simulink library "Kitchen_Lib"  (R2023a)
settings: Solver=VariableStepAuto  StartTime=0.0  StopTime=10.0  RelTol=1e-3  EnableMultiTasking=on
undefined symbols (not defined in the file): Kitc_BusTyp_P, Kitc_BusTypSkyr_C, Kitc_ColrLedColrls_C, Kitc_ColrLedGrn_C, Kitc_ColrLedRed_C, Kitc_ColrLedYlw_C, Kitc_StDgnWtrTank_C, Kitc_StElecPlugScktOffByClmp50_P, Kitc_StsDlyBlink_C, Kitc_StsErrBlink_C, Kitc_StsFctAcvn_P, Kitc_StsInfoBlink_C, Kitc_StsKitchnOffAutoIgOff_P, Kitc_StsKitchnOffBySwt_P, Kitc_StsKitchnOffDoorLockd_P, Kitc_StsKitchnOffIgOff_P, Kitc_StsKitchnOffUv_P, Kitc_StsKitchnOnBySwt_P, Kitc_StsKitchnOnNVM_P, Kitc_StsLedOff_C, Kitc_StsLedOn_C, Kitc_StsLrgCnsAcv_P, Kitc_StTrfrAnSwtInstd_P, Kitc_StTrfrSwtInstd_P, Kitc_TiKitcRefgtrOffDly_P, Kitc_ULowrThdBat_C, Kitc_UUpprThdBat_C, Kitc_ValFalse_C, Kitc_ValPwmFreq2_C, Kitc_ValPwmFreq_C, Kitc_ValTrue_C
libraries: MAN_Library x50, E2E_Lib x3
(part 1 of 13)
settings Model: Creator=l4521  LastModifiedBy=u29w13
settings SolverCC: AlgebraicLoopSolver=TrustRegion
settings DataIOCC: LimitDataPoints=on  ReturnWorkspaceOutputs=off
settings OptimizationCC: LifeSpan=inf
settings DebuggingCC: UnconnectedInputMsg=warning  UnconnectedOutputMsg=warning  UnconnectedLineMsg=warning  AllowSymbolicDim=off  SFUnexpectedBacktrackingDiag=warning  SFNoUnconditionalDefaultTransitionDiag=warning  SFExecutionAtInitializationDiag=none  ArithmeticOperatorsInVariantConditions=warning
settings ModelReferenceCC: EnableRefExpFcnMdlSchedulingChecks=on  PropagateSignalLabelsOutOfModel=off
settings SFSimCC: SimUseLocalCustomCode=off  CustomCodeUndefinedFunction=UseInterfaceOnly
settings RTWCC: RTWUseLocalCustomCode=off
settings CodeAppCC: StateflowObjectComments=on
settings GRTTargetCC: TargetLangStandard=C89/C90 (ANSI)
settings ConfigComp: CovMetricSettings=dw  CovSaveCumulativeToWorkspaceVar=on  CovSaveSingleToWorkspaceVar=on  CovExternalEMLEnable=off

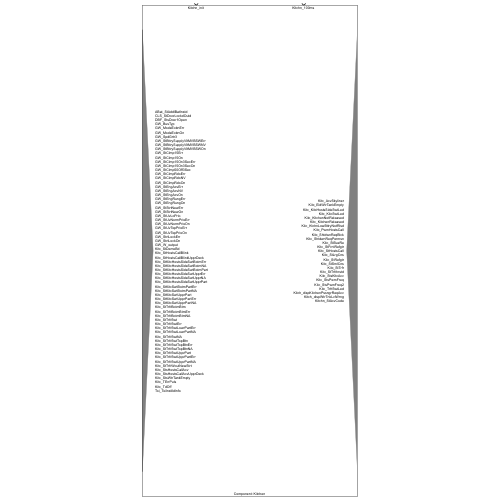
[thumbnail: Simulink's stored preview of the top-level diagram]
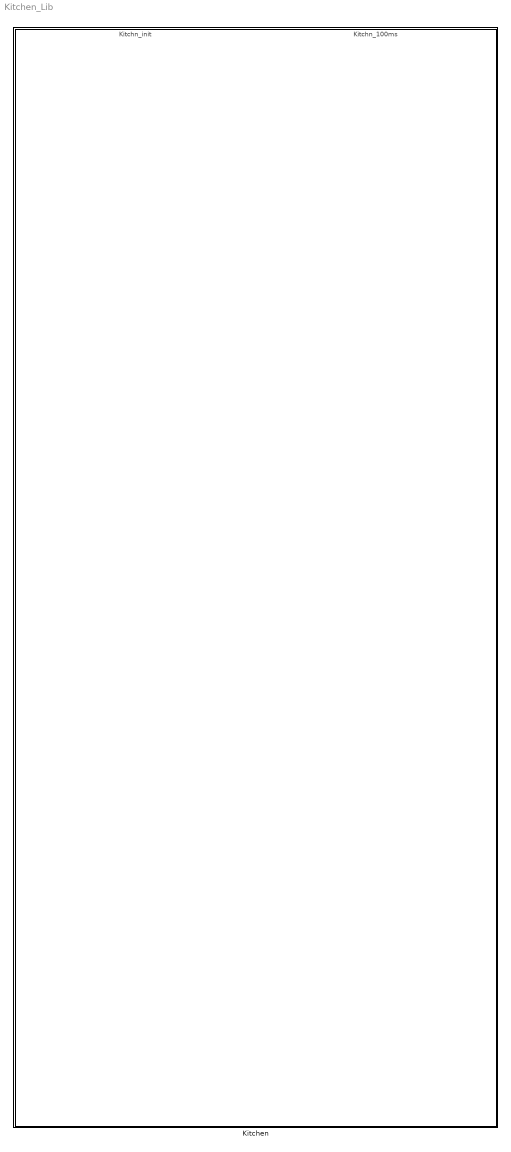
== system Kitchen_Lib ==
  Kitchen : Subsystem  mask(SW Component){}
      settings: MoveFcn=% evalin(get_param(bdroot, 'ModelWorkspace'), get_param(gcb, 'MaskInitialization'));
      mask Display:
      | % SWComponent_mask MaskDisplayStr for SWComponent block
      | %
      | %
      | 
      | % Copyright (c) AVL Software and Functions GmbH 2013
      | % $Revision: 1.42 $, $Date: 2019/08/13 04:53:27UTC $ by $Author: Urlhardt Franz RGB (urlhardf) $
      | 
      | % Calls:
      | 
      | % MaskVersion is used in sl_updateModelTemplate.
      | % $MaskVersion: 1$ % Version must be an integer
      | 
      | ShortName = get_param(gcb,'Name');
      | 
      | % Get inports of function cals
      | inports = find_system(gcb,'SearchDepth',1, 'FollowLinks','on', 'LookUnderMasks','all', 'BlockType','Inport');
      | FcArray = get_param(inports ,'Name');
      | FcXPos = ((1:6)-0.5)/length(FcArray);
      | FcArray(end+1:6) = {''};
      | 
      | % Look for other SW components 1 level below current block
      | SWComponents = find_system(gcb, 'SearchDepth',1, 'FollowLinks','on','LookUnderMasks','all','RegExp','on', 'MaskType','SW Component*');
      | % Remove current block from search results
      | SWComponents(ismember(SWComponents,gcb)) = [];
      | 
      | % A component is a level 3 component if there are no other SW Components below
      | isLevel3 = isempty(SWComponents);
      | 
      | 
      | if isLevel3
      |     % Level 3, Signals form ExtInp and ExtOut blocks
      |     ExtInp = find_system(gcb, 'SearchDepth',inf, 'FollowLinks','on','LookUnderMasks','all', 'MaskType','ExtInp ( AVLib TM )');
      |     ExtOut = find_system(gcb, 'SearchDepth',inf, 'FollowLinks','on','LookUnderMasks','all', 'MaskType','ExtOut ( AVLib TM )');
      | 
      |     Inputs = unique(get_param(ExtInp,'Signal'));
      |     Outputs = unique(get_param(ExtOut,'Signal'));
      | 
      |     %=> No AVLib
      |     if isempty(ExtInp) && isempty(ExtOut);
      |         DSRead = find_system(gcb, 'SearchDepth',2, 'FollowLinks','on','LookUnderMasks','all','BlockType','DataStoreRead');
      |         DSWrite = find_system(gcb, 'SearchDepth',2, 'FollowLinks','on','LookUnderMasks','all','BlockType','DataStoreWrite');
      |         Inputs = unique(get_param(DSRead,'DataStoreName'));
      |         Outputs = unique(get_param(DSWrite,'DataStoreName'));
      |     end
      | 
      |     InpArray = sprintf('%s\n',Inputs{:});
      | 
      |     % Remove last newline character
      |     if ~isempty(Inputs), InpArray(end) = []; end
      | 
      |     OutArray = sprintf('%s\n',Outputs{:});
      |     % Remove last newline character
      |     if ~isempty(Outputs),OutArray(end) = []; end
      | 
      | else
      |     % Level 1/Level 2, get other SWComponents
      |     Comps = get_param(SWComponents,'Name');
      |     CompsArray = sprintf('%s\n',Comps{:});
      |     if ~isempty(Comps), CompsArray(end) = []; end
      | end
      | 
      | 
      | %% Mask
      | % Triangles
      | patch( [0 0.05 0 nan 1 0.95 1],[0.95 0.5 0.05 nan 0.95 0.5 0.05], 0.5*[1 1 1] );
      | 
      | % Names of function calls
      | for i = 1:6
      |     text(FcXPos(i), 1, FcArray{i}, 'HorizontalAlignment','center',  'VerticalAlignment','top'  );
      | end
      | 
      | if isLevel3
      |     % Level 3, display signals of ExtInp and ExtOut blocks
      |     text(0.06, 0.5, InpArray, 'HorizontalAlignment','left',  'VerticalAlignment','middle' );
      |     text(0.94, 0.5, OutArray, 'HorizontalAlignment','right', 'VerticalAlignment','middle' );
      |     text(0.5, 0.0, ['Component: ',ShortName], 'HorizontalAlignment','center', 'VerticalAlignment','bottom' );
      | else
      |     % Level 1/ Level 2, display names of other components below mask
      |     text(0.5, 0.5, CompsArray, 'HorizontalAlignment','center',  'VerticalAlignment','middle' );
      |     text(0.5, 0.0, ['Component: ',ShortName], 'HorizontalAlignment','center', 'VerticalAlignment','bottom' );
      | end

== system Kitchen_Lib/Kitchen ==
  Kitchn_init : Inport
  Kitchn_100ms : Inport  Port=2
  100ms : Subsystem  TreatAsAtomicUnit=on
      settings: RTWSystemCode=Inline
  init : Subsystem  TreatAsAtomicUnit=on
      settings: RTWSystemCode=Inline
  wires:
  Kitchn_100ms/1 -> 100ms/Trigger  "Kitchn_100ms"
  Kitchn_init/1 -> init/Trigger  "Kitchn_init"

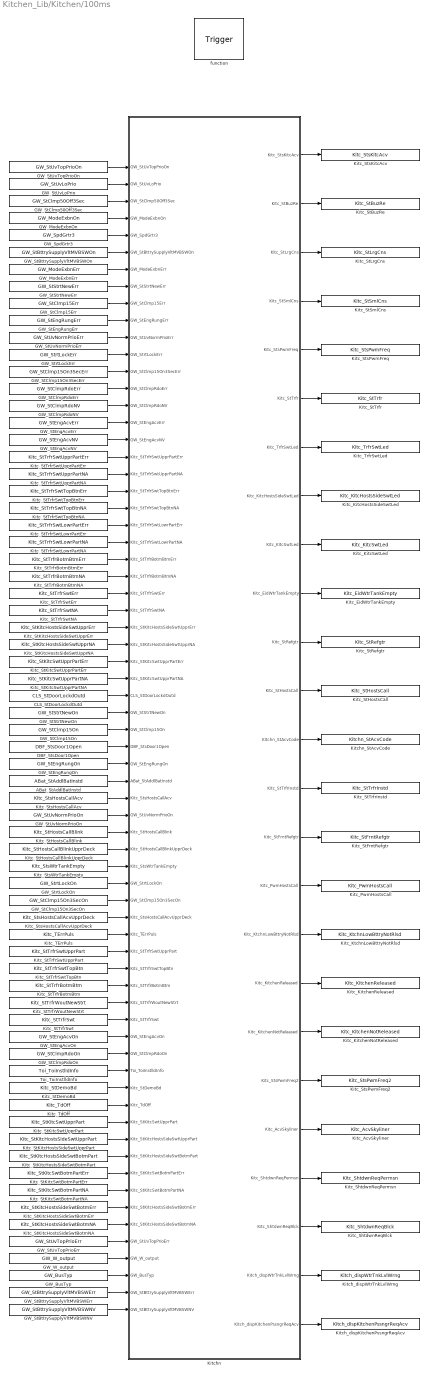
== system Kitchen_Lib/Kitchen/100ms ==
  function : TriggerPort  TriggerType=function-call  VariantControl=(inherit)
  ABat_StAddlBatInstd : DataStoreRead  DataStoreName=ABat_StAddlBatInstd  IndexOptions=Index vector (dialog)  Indices=1  OutputSizes=1
  CLS_StDoorLockdOutd : DataStoreRead  DataStoreName=CLS_StDoorLockdOutd  IndexOptions=Index vector (dialog)  Indices=1  OutputSizes=1
  DBF_StsDoor1Open : DataStoreRead  DataStoreName=DBF_StsDoor1Open  IndexOptions=Index vector (dialog)  Indices=1  OutputSizes=1
  GW_BusTyp : DataStoreRead  DataStoreName=GW_BusTyp  IndexOptions=Index vector (dialog)  Indices=1  OutputSizes=1
  GW_ModeExbnErr : DataStoreRead  DataStoreName=GW_ModeExbnErr  IndexOptions=Index vector (dialog)  Indices=1  OutputSizes=1
  "GW_ModeExbnOn " : DataStoreRead  DataStoreName=GW_ModeExbnOn  IndexOptions=Index vector (dialog)  Indices=1  OutputSizes=1
  GW_SpdGrtr3 : DataStoreRead  DataStoreName=GW_SpdGrtr3  IndexOptions=Index vector (dialog)  Indices=1  OutputSizes=1
  GW_StBttrySupplyVltMVBSWErr : DataStoreRead  DataStoreName=GW_StBttrySupplyVltMVBSWErr  IndexOptions=Index vector (dialog)  Indices=1  OutputSizes=1
  GW_StBttrySupplyVltMVBSWNV : DataStoreRead  DataStoreName=GW_StBttrySupplyVltMVBSWNV  IndexOptions=Index vector (dialog)  Indices=1  OutputSizes=1
  "GW_StBttrySupplyVltMVBSWOn " : DataStoreRead  DataStoreName=GW_StBttrySupplyVltMVBSWOn  IndexOptions=Index vector (dialog)  Indices=1  OutputSizes=1
  GW_StClmp15Err : DataStoreRead  DataStoreName=GW_StClmp15Err  IndexOptions=Index vector (dialog)  Indices=1  OutputSizes=1
  GW_StClmp15On : DataStoreRead  DataStoreName=GW_StClmp15On  IndexOptions=Index vector (dialog)  Indices=1  OutputSizes=1
  GW_StClmp15On3SecErr : DataStoreRead  DataStoreName=GW_StClmp15On3SecErr  IndexOptions=Index vector (dialog)  Indices=1  OutputSizes=1
  "GW_StClmp15On3SecOn " : DataStoreRead  DataStoreName=GW_StClmp15On3SecOn  IndexOptions=Index vector (dialog)  Indices=1  OutputSizes=1
  "GW_StClmp50Off3Sec " : DataStoreRead  DataStoreName=GW_StClmp50Off3Sec  IndexOptions=Index vector (dialog)  Indices=1  OutputSizes=1
  GW_StClmpRdoErr : DataStoreRead  DataStoreName=GW_StClmpRdoErr  IndexOptions=Index vector (dialog)  Indices=1  OutputSizes=1
  GW_StClmpRdoNV : DataStoreRead  DataStoreName=GW_StClmpRdoNV  IndexOptions=Index vector (dialog)  Indices=1  OutputSizes=1
  GW_StClmpRdoOn : DataStoreRead  DataStoreName=GW_StClmpRdoOn  IndexOptions=Index vector (dialog)  Indices=1  OutputSizes=1
  GW_StEngAcvErr : DataStoreRead  DataStoreName=GW_StEngAcvErr  IndexOptions=Index vector (dialog)  Indices=1  OutputSizes=1
  GW_StEngAcvNV : DataStoreRead  DataStoreName=GW_StEngAcvNV  IndexOptions=Index vector (dialog)  Indices=1  OutputSizes=1
  "GW_StEngAcvOn " : DataStoreRead  DataStoreName=GW_StEngAcvOn  IndexOptions=Index vector (dialog)  Indices=1  OutputSizes=1
  GW_StEngRungErr : DataStoreRead  DataStoreName=GW_StEngRungErr  IndexOptions=Index vector (dialog)  Indices=1  OutputSizes=1
  GW_StEngRungOn : DataStoreRead  DataStoreName=GW_StEngRungOn  IndexOptions=Index vector (dialog)  Indices=1  OutputSizes=1
  GW_StStrtNewErr : DataStoreRead  DataStoreName=GW_StStrtNewErr  IndexOptions=Index vector (dialog)  Indices=1  OutputSizes=1
  "GW_StStrtNewOn " : DataStoreRead  DataStoreName=GW_StStrtNewOn  IndexOptions=Index vector (dialog)  Indices=1  OutputSizes=1
  GW_StUvLoPrio : DataStoreRead  DataStoreName=GW_StUvLoPrio  IndexOptions=Index vector (dialog)  Indices=1  OutputSizes=1
  GW_StUvNormPrioErr : DataStoreRead  DataStoreName=GW_StUvNormPrioErr  IndexOptions=Index vector (dialog)  Indices=1  OutputSizes=1
  "GW_StUvNormPrioOn " : DataStoreRead  DataStoreName=GW_StUvNormPrioOn  IndexOptions=Index vector (dialog)  Indices=1  OutputSizes=1
  GW_StUvTopPrioErr : DataStoreRead  DataStoreName=GW_StUvTopPrioErr  IndexOptions=Index vector (dialog)  Indices=1  OutputSizes=1
  GW_StUvTopPrioOn : DataStoreRead  DataStoreName=GW_StUvTopPrioOn  IndexOptions=Index vector (dialog)  Indices=1  OutputSizes=1
  GW_StrtLockErr : DataStoreRead  DataStoreName=GW_StrtLockErr  IndexOptions=Index vector (dialog)  Indices=1  OutputSizes=1
  "GW_StrtLockOn " : DataStoreRead  DataStoreName=GW_StrtLockOn  IndexOptions=Index vector (dialog)  Indices=1  OutputSizes=1
  GW_W_output : DataStoreRead  DataStoreName=GW_W_output  IndexOptions=Index vector (dialog)  Indices=1  OutputSizes=1
  Kitc_AcvSkyliner : DataStoreWrite  DataStoreName=Kitc_AcvSkyliner  IndexOptions=Index vector (dialog)  Indices=1  OutputSizes=1
  Kitc_EidWtrTankEmpty : DataStoreWrite  DataStoreName=Kitc_EidWtrTankEmpty  IndexOptions=Index vector (dialog)  Indices=1  OutputSizes=1
  Kitc_KitcHostsSideSwtLed : DataStoreWrite  DataStoreName=Kitc_KitcHostsSideSwtLed  IndexOptions=Index vector (dialog)  Indices=1  OutputSizes=1
  Kitc_KitcSwtLed : DataStoreWrite  DataStoreName=Kitc_KitcSwtLed  IndexOptions=Index vector (dialog)  Indices=1  OutputSizes=1
  Kitc_KitchenNotReleased : DataStoreWrite  DataStoreName=Kitc_KitchenNotReleased  IndexOptions=Index vector (dialog)  Indices=1  OutputSizes=1
  Kitc_KitchenReleased : DataStoreWrite  DataStoreName=Kitc_KitchenReleased  IndexOptions=Index vector (dialog)  Indices=1  OutputSizes=1
  Kitc_KtchnLowBttryNotRlsd : DataStoreWrite  DataStoreName=Kitc_KtchnLowBttryNotRlsd  IndexOptions=Index vector (dialog)  Indices=1  OutputSizes=1
  Kitc_PwmHostsCall : DataStoreWrite  DataStoreName=Kitc_PwmHostsCall  IndexOptions=Index vector (dialog)  Indices=1  OutputSizes=1
  Kitc_ShtdwnReqBlck : DataStoreWrite  DataStoreName=Kitc_ShtdwnReqBlck  IndexOptions=Index vector (dialog)  Indices=1  OutputSizes=1
  Kitc_ShtdwnReqPermsn : DataStoreWrite  DataStoreName=Kitc_ShtdwnReqPermsn  IndexOptions=Index vector (dialog)  Indices=1  OutputSizes=1
  Kitc_StBuzRe : DataStoreWrite  DataStoreName=Kitc_StBuzRe  IndexOptions=Index vector (dialog)  Indices=1  OutputSizes=1
  Kitc_StDemoBd : DataStoreRead  DataStoreName=Kitc_StDemoBd  IndexOptions=Index vector (dialog)  Indices=1  OutputSizes=1
  "Kitc_StFrntRefgtr " : DataStoreWrite  DataStoreName=Kitc_StFrntRefgtr  IndexOptions=Index vector (dialog)  Indices=1  OutputSizes=1
  Kitc_StHostsCall : DataStoreWrite  DataStoreName=Kitc_StHostsCall  IndexOptions=Index vector (dialog)  Indices=1  OutputSizes=1
  Kitc_StHostsCallBlink : DataStoreRead  DataStoreName=Kitc_StHostsCallBlink  IndexOptions=Index vector (dialog)  Indices=1  OutputSizes=1
  Kitc_StHostsCallBlinkUpprDeck : DataStoreRead  DataStoreName=Kitc_StHostsCallBlinkUpprDeck  IndexOptions=Index vector (dialog)  Indices=1  OutputSizes=1
  Kitc_StKitcHostsSideSwtBotmErr : DataStoreRead  DataStoreName=Kitc_StKitcHostsSideSwtBotmErr  IndexOptions=Index vector (dialog)  Indices=1  OutputSizes=1
  Kitc_StKitcHostsSideSwtBotmNA : DataStoreRead  DataStoreName=Kitc_StKitcHostsSideSwtBotmNA  IndexOptions=Index vector (dialog)  Indices=1  OutputSizes=1
  Kitc_StKitcHostsSideSwtBotmPart : DataStoreRead  DataStoreName=Kitc_StKitcHostsSideSwtBotmPart  IndexOptions=Index vector (dialog)  Indices=1  OutputSizes=1
  Kitc_StKitcHostsSideSwtUpprErr : DataStoreRead  DataStoreName=Kitc_StKitcHostsSideSwtUpprErr  IndexOptions=Index vector (dialog)  Indices=1  OutputSizes=1
  Kitc_StKitcHostsSideSwtUpprNA : DataStoreRead  DataStoreName=Kitc_StKitcHostsSideSwtUpprNA  IndexOptions=Index vector (dialog)  Indices=1  OutputSizes=1
  Kitc_StKitcHostsSideSwtUpprPart : DataStoreRead  DataStoreName=Kitc_StKitcHostsSideSwtUpprPart  IndexOptions=Index vector (dialog)  Indices=1  OutputSizes=1
  Kitc_StKitcSwtBotmPartErr : DataStoreRead  DataStoreName=Kitc_StKitcSwtBotmPartErr  IndexOptions=Index vector (dialog)  Indices=1  OutputSizes=1
  Kitc_StKitcSwtBotmPartNA : DataStoreRead  DataStoreName=Kitc_StKitcSwtBotmPartNA  IndexOptions=Index vector (dialog)  Indices=1  OutputSizes=1
  Kitc_StKitcSwtUpprPart : DataStoreRead  DataStoreName=Kitc_StKitcSwtUpprPart  IndexOptions=Index vector (dialog)  Indices=1  OutputSizes=1
  Kitc_StKitcSwtUpprPartErr : DataStoreRead  DataStoreName=Kitc_StKitcSwtUpprPartErr  IndexOptions=Index vector (dialog)  Indices=1  OutputSizes=1
  Kitc_StKitcSwtUpprPartNA : DataStoreRead  DataStoreName=Kitc_StKitcSwtUpprPartNA  IndexOptions=Index vector (dialog)  Indices=1  OutputSizes=1
  Kitc_StLrgCns : DataStoreWrite  DataStoreName=Kitc_StLrgCns  IndexOptions=Index vector (dialog)  Indices=1  OutputSizes=1
  Kitc_StRefgtr : DataStoreWrite  DataStoreName=Kitc_StRefgtr  IndexOptions=Index vector (dialog)  Indices=1  OutputSizes=1
  Kitc_StSmlCns : DataStoreWrite  DataStoreName=Kitc_StSmlCns  IndexOptions=Index vector (dialog)  Indices=1  OutputSizes=1
  Kitc_StTrfr : DataStoreWrite  DataStoreName=Kitc_StTrfr  IndexOptions=Index vector (dialog)  Indices=1  OutputSizes=1
  Kitc_StTrfrBotmBtm : DataStoreRead  DataStoreName=Kitc_StTrfrBotmBtm  IndexOptions=Index vector (dialog)  Indices=1  OutputSizes=1
  Kitc_StTrfrBotmBtmErr : DataStoreRead  DataStoreName=Kitc_StTrfrBotmBtmErr  IndexOptions=Index vector (dialog)  Indices=1  OutputSizes=1
  Kitc_StTrfrBotmBtmNA : DataStoreRead  DataStoreName=Kitc_StTrfrBotmBtmNA  IndexOptions=Index vector (dialog)  Indices=1  OutputSizes=1
  Kitc_StTrfrInstd : DataStoreWrite  DataStoreName=Kitc_StTrfrInstd  IndexOptions=Index vector (dialog)  Indices=1  OutputSizes=1
  "Kitc_StTrfrSwt " : DataStoreRead  DataStoreName=Kitc_StTrfrSwt  IndexOptions=Index vector (dialog)  Indices=1  OutputSizes=1
  Kitc_StTrfrSwtErr : DataStoreRead  DataStoreName=Kitc_StTrfrSwtErr  IndexOptions=Index vector (dialog)  Indices=1  OutputSizes=1
  Kitc_StTrfrSwtLowrPartErr : DataStoreRead  DataStoreName=Kitc_StTrfrSwtLowrPartErr  IndexOptions=Index vector (dialog)  Indices=1  OutputSizes=1
  Kitc_StTrfrSwtLowrPartNA : DataStoreRead  DataStoreName=Kitc_StTrfrSwtLowrPartNA  IndexOptions=Index vector (dialog)  Indices=1  OutputSizes=1
  Kitc_StTrfrSwtNA : DataStoreRead  DataStoreName=Kitc_StTrfrSwtNA  IndexOptions=Index vector (dialog)  Indices=1  OutputSizes=1
  Kitc_StTrfrSwtTopBtn : DataStoreRead  DataStoreName=Kitc_StTrfrSwtTopBtn  IndexOptions=Index vector (dialog)  Indices=1  OutputSizes=1
  Kitc_StTrfrSwtTopBtnErr : DataStoreRead  DataStoreName=Kitc_StTrfrSwtTopBtnErr  IndexOptions=Index vector (dialog)  Indices=1  OutputSizes=1
  Kitc_StTrfrSwtTopBtnNA : DataStoreRead  DataStoreName=Kitc_StTrfrSwtTopBtnNA  IndexOptions=Index vector (dialog)  Indices=1  OutputSizes=1
  Kitc_StTrfrSwtUpprPart : DataStoreRead  DataStoreName=Kitc_StTrfrSwtUpprPart  IndexOptions=Index vector (dialog)  Indices=1  OutputSizes=1
  Kitc_StTrfrSwtUpprPartErr : DataStoreRead  DataStoreName=Kitc_StTrfrSwtUpprPartErr  IndexOptions=Index vector (dialog)  Indices=1  OutputSizes=1
  Kitc_StTrfrSwtUpprPartNA : DataStoreRead  DataStoreName=Kitc_StTrfrSwtUpprPartNA  IndexOptions=Index vector (dialog)  Indices=1  OutputSizes=1
  Kitc_StTrfrWoutNewStrt : DataStoreRead  DataStoreName=Kitc_StTrfrWoutNewStrt  IndexOptions=Index vector (dialog)  Indices=1  OutputSizes=1
  Kitc_StsHostsCallAcv : DataStoreRead  DataStoreName=Kitc_StsHostsCallAcv  IndexOptions=Index vector (dialog)  Indices=1  OutputSizes=1
  Kitc_StsHostsCallAcvUpprDeck : DataStoreRead  DataStoreName=Kitc_StsHostsCallAcvUpprDeck  IndexOptions=Index vector (dialog)  Indices=1  OutputSizes=1
  Kitc_StsKitcAcv : DataStoreWrite  DataStoreName=Kitc_StsKitcAcv  IndexOptions=Index vector (dialog)  Indices=1  OutputSizes=1
  Kitc_StsPwmFreq : DataStoreWrite  DataStoreName=Kitc_StsPwmFreq  IndexOptions=Index vector (dialog)  Indices=1  OutputSizes=1
  Kitc_StsPwmFreq2 : DataStoreWrite  DataStoreName=Kitc_StsPwmFreq2  IndexOptions=Index vector (dialog)  Indices=1  OutputSizes=1
  Kitc_StsWtrTankEmpty : DataStoreRead  DataStoreName=Kitc_StsWtrTankEmpty  IndexOptions=Index vector (dialog)  Indices=1  OutputSizes=1
  Kitc_TErrPuls : DataStoreRead  DataStoreName=Kitc_TErrPuls  IndexOptions=Index vector (dialog)  Indices=1  OutputSizes=1
  Kitc_TdOff : DataStoreRead  DataStoreName=Kitc_TdOff  IndexOptions=Index vector (dialog)  Indices=1  OutputSizes=1
  Kitc_TrfrSwtLed : DataStoreWrite  DataStoreName=Kitc_TrfrSwtLed  IndexOptions=Index vector (dialog)  Indices=1  OutputSizes=1
  Kitch_dispKitchenPssngrReqAcv : DataStoreWrite  DataStoreName=Kitch_dispKitchenPssngrReqAcv  IndexOptions=Index vector (dialog)  Indices=1  OutputSizes=1
  Kitch_dispWtrTnkLvlWrng : DataStoreWrite  DataStoreName=Kitch_dispWtrTnkLvlWrng  IndexOptions=Index vector (dialog)  Indices=1  OutputSizes=1
  Kitchn : Subsystem
  Kitchn_StAcvCode : DataStoreWrite  DataStoreName=Kitchn_StAcvCode  IndexOptions=Index vector (dialog)  Indices=1  OutputSizes=1
  Toi_ToiInstlldInfo : DataStoreRead  DataStoreName=Toi_ToiInstlldInfo  IndexOptions=Index vector (dialog)  Indices=1  OutputSizes=1
  wires:
  Kitchn/25(Kitch_dispKitchenPssngrReqAcv) -> Kitch_dispKitchenPssngrReqAcv/1
  Kitchn/24(Kitch_dispWtrTnkLvlWrng) -> Kitch_dispWtrTnkLvlWrng/1
  Kitchn/23(Kitc_ShtdwnReqBlck) -> Kitc_ShtdwnReqBlck/1
  Kitchn/22(Kitc_ShtdwnReqPermsn) -> Kitc_ShtdwnReqPermsn/1
  Kitchn/21(Kitc_AcvSkyliner) -> Kitc_AcvSkyliner/1
  Kitchn/20(Kitc_StsPwmFreq2) -> Kitc_StsPwmFreq2/1
  Kitchn/19(Kitc_KitchenNotReleased) -> Kitc_KitchenNotReleased/1
  Kitchn/18(Kitc_KitchenReleased) -> Kitc_KitchenReleased/1
  Kitchn/17(Kitc_KtchnLowBttryNotRlsd) -> Kitc_KtchnLowBttryNotRlsd/1
  Kitchn/16(Kitc_PwmHostsCall) -> Kitc_PwmHostsCall/1
  Kitchn/15("Kitc_StFrntRefgtr ") -> "Kitc_StFrntRefgtr "/1
  Kitchn/14(Kitc_StTrfrInstd) -> Kitc_StTrfrInstd/1
  Kitchn/13(Kitchn_StAcvCode) -> Kitchn_StAcvCode/1
  Kitchn/12(Kitc_StHostsCall) -> Kitc_StHostsCall/1
  Kitchn/11(Kitc_StRefgtr) -> Kitc_StRefgtr/1
  Kitchn/10(Kitc_EidWtrTankEmpty) -> Kitc_EidWtrTankEmpty/1
  Kitchn/9(Kitc_KitcSwtLed) -> Kitc_KitcSwtLed/1
  Kitchn/8(Kitc_KitcHostsSideSwtLed) -> Kitc_KitcHostsSideSwtLed/1
  Kitchn/7(Kitc_TrfrSwtLed) -> Kitc_TrfrSwtLed/1
  Kitchn/6(Kitc_StTrfr) -> Kitc_StTrfr/1
  Kitchn/5(Kitc_StsPwmFreq) -> Kitc_StsPwmFreq/1
  Kitchn/4(Kitc_StSmlCns) -> Kitc_StSmlCns/1
  Kitchn/3(Kitc_StLrgCns) -> Kitc_StLrgCns/1
  Kitchn/2(Kitc_StBuzRe) -> Kitc_StBuzRe/1
  Kitchn/1(Kitc_StsKitcAcv) -> Kitc_StsKitcAcv/1
  GW_StBttrySupplyVltMVBSWNV/1 -> Kitchn/68(GW_StBttrySupplyVltMVBSWNV)
  GW_StBttrySupplyVltMVBSWErr/1 -> Kitchn/67(GW_StBttrySupplyVltMVBSWErr)
  GW_BusTyp/1 -> Kitchn/66(GW_BusTyp)
  GW_W_output/1 -> Kitchn/65(GW_W_output)
  GW_StUvTopPrioErr/1 -> Kitchn/64(GW_StUvTopPrioErr)
  Kitc_StKitcHostsSideSwtBotmNA/1 -> Kitchn/63(Kitc_StKitcHostsSideSwtBotmNA)
  Kitc_StKitcHostsSideSwtBotmErr/1 -> Kitchn/62(Kitc_StKitcHostsSideSwtBotmErr)
  Kitc_StKitcSwtBotmPartNA/1 -> Kitchn/61(Kitc_StKitcSwtBotmPartNA)
  Kitc_StKitcSwtBotmPartErr/1 -> Kitchn/60(Kitc_StKitcSwtBotmPartErr)
  Kitc_StKitcHostsSideSwtBotmPart/1 -> Kitchn/59(Kitc_StKitcHostsSideSwtBotmPart)
  Kitc_StKitcHostsSideSwtUpprPart/1 -> Kitchn/58(Kitc_StKitcHostsSideSwtUpprPart)
  Kitc_StKitcSwtUpprPart/1 -> Kitchn/57(Kitc_StKitcSwtUpprPart)
  Kitc_TdOff/1 -> Kitchn/56(Kitc_TdOff)
  Kitc_StDemoBd/1 -> Kitchn/55(Kitc_StDemoBd)
  Toi_ToiInstlldInfo/1 -> Kitchn/54(Toi_ToiInstlldInfo)
  GW_StClmpRdoOn/1 -> Kitchn/53(GW_StClmpRdoOn)
  "GW_StEngAcvOn "/1 -> Kitchn/52("GW_StEngAcvOn ")
  "Kitc_StTrfrSwt "/1 -> Kitchn/51("Kitc_StTrfrSwt ")
  Kitc_StTrfrWoutNewStrt/1 -> Kitchn/50(Kitc_StTrfrWoutNewStrt)
  Kitc_StTrfrBotmBtm/1 -> Kitchn/49(Kitc_StTrfrBotmBtm)
  Kitc_StTrfrSwtTopBtn/1 -> Kitchn/48(Kitc_StTrfrSwtTopBtn)
  Kitc_StTrfrSwtUpprPart/1 -> Kitchn/47(Kitc_StTrfrSwtUpprPart)
  Kitc_TErrPuls/1 -> Kitchn/46(Kitc_TErrPuls)
  Kitc_StsHostsCallAcvUpprDeck/1 -> Kitchn/45(Kitc_StsHostsCallAcvUpprDeck)
  "GW_StClmp15On3SecOn "/1 -> Kitchn/44("GW_StClmp15On3SecOn ")
  "GW_StrtLockOn "/1 -> Kitchn/43("GW_StrtLockOn ")
  Kitc_StsWtrTankEmpty/1 -> Kitchn/42(Kitc_StsWtrTankEmpty)
  Kitc_StHostsCallBlinkUpprDeck/1 -> Kitchn/41(Kitc_StHostsCallBlinkUpprDeck)
  Kitc_StHostsCallBlink/1 -> Kitchn/40(Kitc_StHostsCallBlink)
  "GW_StUvNormPrioOn "/1 -> Kitchn/39("GW_StUvNormPrioOn ")
  Kitc_StsHostsCallAcv/1 -> Kitchn/38(Kitc_StsHostsCallAcv)
  ABat_StAddlBatInstd/1 -> Kitchn/37(ABat_StAddlBatInstd)
  GW_StEngRungOn/1 -> Kitchn/36(GW_StEngRungOn)
  DBF_StsDoor1Open/1 -> Kitchn/35(DBF_StsDoor1Open)
  GW_StClmp15On/1 -> Kitchn/34(GW_StClmp15On)
  "GW_StStrtNewOn "/1 -> Kitchn/33("GW_StStrtNewOn ")
  CLS_StDoorLockdOutd/1 -> Kitchn/32(CLS_StDoorLockdOutd)
  Kitc_StKitcSwtUpprPartNA/1 -> Kitchn/31(Kitc_StKitcSwtUpprPartNA)
  Kitc_StKitcSwtUpprPartErr/1 -> Kitchn/30(Kitc_StKitcSwtUpprPartErr)
  Kitc_StKitcHostsSideSwtUpprNA/1 -> Kitchn/29(Kitc_StKitcHostsSideSwtUpprNA)
  Kitc_StKitcHostsSideSwtUpprErr/1 -> Kitchn/28(Kitc_StKitcHostsSideSwtUpprErr)
  Kitc_StTrfrSwtNA/1 -> Kitchn/27(Kitc_StTrfrSwtNA)
  Kitc_StTrfrSwtErr/1 -> Kitchn/26(Kitc_StTrfrSwtErr)
  Kitc_StTrfrBotmBtmNA/1 -> Kitchn/25(Kitc_StTrfrBotmBtmNA)
  Kitc_StTrfrBotmBtmErr/1 -> Kitchn/24(Kitc_StTrfrBotmBtmErr)
  Kitc_StTrfrSwtLowrPartNA/1 -> Kitchn/23(Kitc_StTrfrSwtLowrPartNA)
  Kitc_StTrfrSwtLowrPartErr/1 -> Kitchn/22(Kitc_StTrfrSwtLowrPartErr)
  Kitc_StTrfrSwtTopBtnNA/1 -> Kitchn/21(Kitc_StTrfrSwtTopBtnNA)
  Kitc_StTrfrSwtTopBtnErr/1 -> Kitchn/20(Kitc_StTrfrSwtTopBtnErr)
  Kitc_StTrfrSwtUpprPartNA/1 -> Kitchn/19(Kitc_StTrfrSwtUpprPartNA)
  Kitc_StTrfrSwtUpprPartErr/1 -> Kitchn/18(Kitc_StTrfrSwtUpprPartErr)
  GW_StEngAcvNV/1 -> Kitchn/17(GW_StEngAcvNV)
  GW_StEngAcvErr/1 -> Kitchn/16(GW_StEngAcvErr)
  GW_StClmpRdoNV/1 -> Kitchn/15(GW_StClmpRdoNV)
  GW_StClmpRdoErr/1 -> Kitchn/14(GW_StClmpRdoErr)
  GW_StClmp15On3SecErr/1 -> Kitchn/13(GW_StClmp15On3SecErr)
  GW_StrtLockErr/1 -> Kitchn/12(GW_StrtLockErr)
  GW_StUvNormPrioErr/1 -> Kitchn/11(GW_StUvNormPrioErr)
  GW_StEngRungErr/1 -> Kitchn/10(GW_StEngRungErr)
  GW_StClmp15Err/1 -> Kitchn/9(GW_StClmp15Err)
  GW_StStrtNewErr/1 -> Kitchn/8(GW_StStrtNewErr)
  GW_ModeExbnErr/1 -> Kitchn/7(GW_ModeExbnErr)
  "GW_StBttrySupplyVltMVBSWOn "/1 -> Kitchn/6("GW_StBttrySupplyVltMVBSWOn ")
  GW_SpdGrtr3/1 -> Kitchn/5(GW_SpdGrtr3)
  "GW_ModeExbnOn "/1 -> Kitchn/4("GW_ModeExbnOn ")
  "GW_StClmp50Off3Sec "/1 -> Kitchn/3("GW_StClmp50Off3Sec ")
  GW_StUvLoPrio/1 -> Kitchn/2(GW_StUvLoPrio)
  GW_StUvTopPrioOn/1 -> Kitchn/1(GW_StUvTopPrioOn)

== system Kitchen_Lib/Kitchen/init ==
  function : TriggerPort  TriggerType=function-call  VariantControl=(inherit)

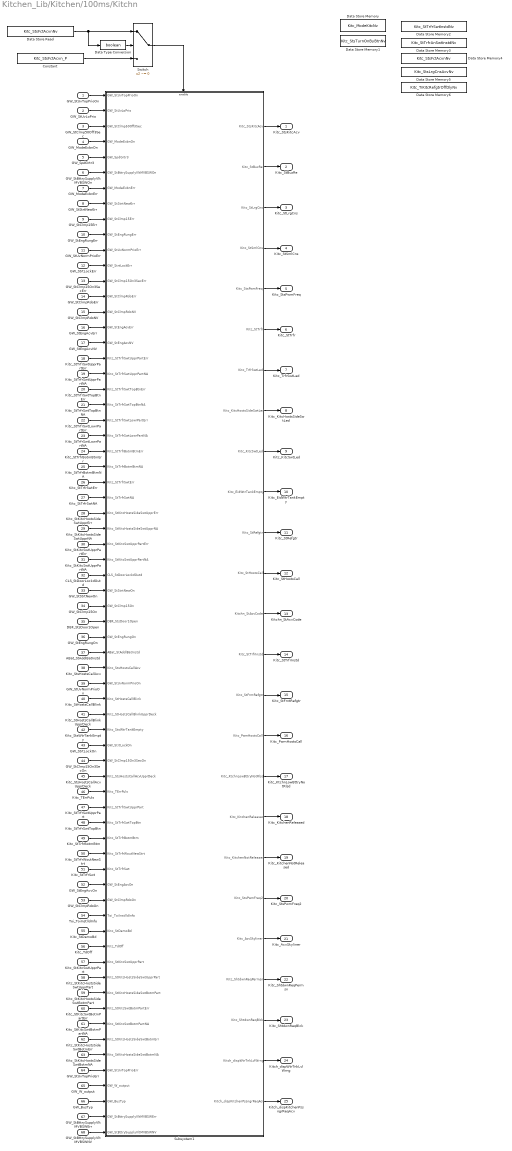
== system Kitchen_Lib/Kitchen/100ms/Kitchn ==
  GW_StUvTopPrioOn : Inport
  GW_StUvLoPrio : Inport  Port=2
  "GW_StClmp50Off3Sec " : Inport  Port=3
  "GW_ModeExbnOn " : Inport  Port=4
  GW_SpdGrtr3 : Inport  Port=5
  "GW_StBttrySupplyVltMVBSWOn " : Inport  Port=6
  GW_ModeExbnErr : Inport  Port=7
  GW_StStrtNewErr : Inport  Port=8
  GW_StClmp15Err : Inport  Port=9
  GW_StEngRungErr : Inport  Port=10
  GW_StUvNormPrioErr : Inport  Port=11
  GW_StrtLockErr : Inport  Port=12
  GW_StClmp15On3SecErr : Inport  Port=13
  GW_StClmpRdoErr : Inport  Port=14
  GW_StClmpRdoNV : Inport  Port=15
  GW_StEngAcvErr : Inport  Port=16
  GW_StEngAcvNV : Inport  Port=17
  Kitc_StTrfrSwtUpprPartErr : Inport  Port=18
  Kitc_StTrfrSwtUpprPartNA : Inport  Port=19
  Kitc_StTrfrSwtTopBtnErr : Inport  Port=20
  Kitc_StTrfrSwtTopBtnNA : Inport  Port=21
  Kitc_StTrfrSwtLowrPartErr : Inport  Port=22
  Kitc_StTrfrSwtLowrPartNA : Inport  Port=23
  Kitc_StTrfrBotmBtmErr : Inport  Port=24
  Kitc_StTrfrBotmBtmNA : Inport  Port=25
  Kitc_StTrfrSwtErr : Inport  Port=26
  Kitc_StTrfrSwtNA : Inport  Port=27
  Kitc_StKitcHostsSideSwtUpprErr : Inport  Port=28
  Kitc_StKitcHostsSideSwtUpprNA : Inport  Port=29
  Kitc_StKitcSwtUpprPartErr : Inport  Port=30
  Kitc_StKitcSwtUpprPartNA : Inport  Port=31
  CLS_StDoorLockdOutd : Inport  Port=32
  "GW_StStrtNewOn " : Inport  Port=33
  GW_StClmp15On : Inport  Port=34
  DBF_StsDoor1Open : Inport  Port=35
  GW_StEngRungOn : Inport  Port=36
  ABat_StAddlBatInstd : Inport  Port=37
  Kitc_StsHostsCallAcv : Inport  Port=38
  "GW_StUvNormPrioOn " : Inport  Port=39
  Kitc_StHostsCallBlink : Inport  Port=40
  Kitc_StHostsCallBlinkUpprDeck : Inport  Port=41
  Kitc_StsWtrTankEmpty : Inport  Port=42
  "GW_StrtLockOn " : Inport  Port=43
  "GW_StClmp15On3SecOn " : Inport  Port=44
  Kitc_StsHostsCallAcvUpprDeck : Inport  Port=45
  Kitc_TErrPuls : Inport  Port=46
  Kitc_StTrfrSwtUpprPart : Inport  Port=47
  Kitc_StTrfrSwtTopBtn : Inport  Port=48
  Kitc_StTrfrBotmBtm : Inport  Port=49
  Kitc_StTrfrWoutNewStrt : Inport  Port=50
  "Kitc_StTrfrSwt " : Inport  Port=51
  "GW_StEngAcvOn " : Inport  Port=52
  GW_StClmpRdoOn : Inport  Port=53
  Toi_ToiInstlldInfo : Inport  Port=54
  Kitc_StDemoBd : Inport  Port=55
  Kitc_TdOff : Inport  Port=56
  Kitc_StKitcSwtUpprPart : Inport  Port=57
  Kitc_StKitcHostsSideSwtUpprPart : Inport  Port=58
  Kitc_StKitcHostsSideSwtBotmPart : Inport  Port=59
  Kitc_StKitcSwtBotmPartErr : Inport  Port=60
  Kitc_StKitcSwtBotmPartNA : Inport  Port=61
  Kitc_StKitcHostsSideSwtBotmErr : Inport  Port=62
  Kitc_StKitcHostsSideSwtBotmNA : Inport  Port=63
  GW_StUvTopPrioErr : Inport  Port=64
  GW_W_output : Inport  Port=65
  GW_BusTyp : Inport  Port=66
  GW_StBttrySupplyVltMVBSWErr : Inport  Port=67
  GW_StBttrySupplyVltMVBSWNV : Inport  Port=68
  Constant : Constant  Value=Kitc_StsFctAcvn_P
  Data Store Memory : DataStoreMemory  DataStoreName=Kitc_ModeKitcNv  ReadBeforeWriteMsg=warning  WriteAfterWriteMsg=warning  WriteAfterReadMsg=warning  ShowAdditionalParam=off
  Data Store Memory1 : DataStoreMemory  DataStoreName=Kitc_StsTurnOnByBtnNv  ReadBeforeWriteMsg=warning  WriteAfterWriteMsg=warning  WriteAfterReadMsg=warning  ShowAdditionalParam=off
  Data Store Memory2 : DataStoreMemory  DataStoreName=Kitc_StTrfrSwtInstdNv  ReadBeforeWriteMsg=warning  WriteAfterWriteMsg=warning  WriteAfterReadMsg=warning  ShowAdditionalParam=off  StateMustResolveToSignalObject=on
  Data Store Memory3 : DataStoreMemory  DataStoreName=Kitc_StTrfrAnSwtInstdNv  ReadBeforeWriteMsg=warning  WriteAfterWriteMsg=warning  WriteAfterReadMsg=warning  ShowAdditionalParam=off  StateMustResolveToSignalObject=on
  Data Store Memory4 : DataStoreMemory  DataStoreName=Kitc_StsFctAcvnNv  ReadBeforeWriteMsg=warning  WriteAfterWriteMsg=warning  WriteAfterReadMsg=warning  ShowAdditionalParam=off  StateMustResolveToSignalObject=on
  Data Store Memory5 : DataStoreMemory  DataStoreName=Kitc_StsLrgCnsAcvNv  ReadBeforeWriteMsg=warning  WriteAfterWriteMsg=warning  WriteAfterReadMsg=warning  ShowAdditionalParam=off  StateMustResolveToSignalObject=on
  Data Store Memory6 : DataStoreMemory  DataStoreName=Kitc_TiKitcRefgtrOffDlyNv  ReadBeforeWriteMsg=warning  WriteAfterWriteMsg=warning  WriteAfterReadMsg=warning  ShowAdditionalParam=off  StateMustResolveToSignalObject=on
  Data Store Read : DataStoreRead  DataStoreName=Kitc_StsFctAcvnNv  IndexOptions=Index vector (dialog)  Indices=1  OutputSizes=1
  Data Type Conversion : DataTypeConversion  OutDataTypeStr=boolean  SaturateOnIntegerOverflow=off  RndMeth=Floor
  Subsystem1 : Subsystem
  Switch : Switch  Criteria=u2 ~= 0  SaturateOnIntegerOverflow=off  InputSameDT=off
  Kitc_StsKitcAcv : Outport
  Kitc_StBuzRe : Outport  Port=2
  Kitc_StLrgCns : Outport  Port=3
  Kitc_StSmlCns : Outport  Port=4
  Kitc_StsPwmFreq : Outport  Port=5
  Kitc_StTrfr : Outport  Port=6
  Kitc_TrfrSwtLed : Outport  Port=7
  Kitc_KitcHostsSideSwtLed : Outport  Port=8
  Kitc_KitcSwtLed : Outport  Port=9
  Kitc_EidWtrTankEmpty : Outport  Port=10
  Kitc_StRefgtr : Outport  Port=11
  Kitc_StHostsCall : Outport  Port=12
  Kitchn_StAcvCode : Outport  Port=13
  Kitc_StTrfrInstd : Outport  Port=14
  "Kitc_StFrntRefgtr " : Outport  Port=15
  Kitc_PwmHostsCall : Outport  Port=16
  Kitc_KtchnLowBttryNotRlsd : Outport  Port=17
  Kitc_KitchenReleased : Outport  Port=18
  Kitc_KitchenNotReleased : Outport  Port=19
  Kitc_StsPwmFreq2 : Outport  Port=20
  Kitc_AcvSkyliner : Outport  Port=21
  Kitc_ShtdwnReqPermsn : Outport  Port=22
  Kitc_ShtdwnReqBlck : Outport  Port=23
  Kitch_dispWtrTnkLvlWrng : Outport  Port=24
  Kitch_dispKitchenPssngrReqAcv : Outport  Port=25
  wires:
  Subsystem1/25(Kitch_dispKitchenPssngrReqAcv) -> Kitch_dispKitchenPssngrReqAcv/1
  Subsystem1/24(Kitch_dispWtrTnkLvlWrng) -> Kitch_dispWtrTnkLvlWrng/1
  Subsystem1/23(Kitc_ShtdwnReqBlck) -> Kitc_ShtdwnReqBlck/1
  Subsystem1/22(Kitc_ShtdwnReqPermsn) -> Kitc_ShtdwnReqPermsn/1
  Subsystem1/21(Kitc_AcvSkyliner) -> Kitc_AcvSkyliner/1
  Subsystem1/20(Kitc_StsPwmFreq2) -> Kitc_StsPwmFreq2/1
  Subsystem1/19(Kitc_KitchenNotReleased) -> Kitc_KitchenNotReleased/1
  Subsystem1/18(Kitc_KitchenReleased) -> Kitc_KitchenReleased/1
  Subsystem1/17(Kitc_KtchnLowBttryNotRlsd) -> Kitc_KtchnLowBttryNotRlsd/1
  Subsystem1/16(Kitc_PwmHostsCall) -> Kitc_PwmHostsCall/1
  Subsystem1/15("Kitc_StFrntRefgtr ") -> "Kitc_StFrntRefgtr "/1
  Subsystem1/14(Kitc_StTrfrInstd) -> Kitc_StTrfrInstd/1
  Subsystem1/13(Kitchn_StAcvCode) -> Kitchn_StAcvCode/1
  Subsystem1/12(Kitc_StHostsCall) -> Kitc_StHostsCall/1
  Subsystem1/11(Kitc_StRefgtr) -> Kitc_StRefgtr/1
  Subsystem1/10(Kitc_EidWtrTankEmpty) -> Kitc_EidWtrTankEmpty/1
  Subsystem1/9(Kitc_KitcSwtLed) -> Kitc_KitcSwtLed/1
  Subsystem1/8(Kitc_KitcHostsSideSwtLed) -> Kitc_KitcHostsSideSwtLed/1
  Subsystem1/7(Kitc_TrfrSwtLed) -> Kitc_TrfrSwtLed/1
  Subsystem1/6(Kitc_StTrfr) -> Kitc_StTrfr/1
  Subsystem1/5(Kitc_StsPwmFreq) -> Kitc_StsPwmFreq/1
  Subsystem1/4(Kitc_StSmlCns) -> Kitc_StSmlCns/1
  Subsystem1/3(Kitc_StLrgCns) -> Kitc_StLrgCns/1
  Subsystem1/2(Kitc_StBuzRe) -> Kitc_StBuzRe/1
  Subsystem1/1(Kitc_StsKitcAcv) -> Kitc_StsKitcAcv/1
  GW_StBttrySupplyVltMVBSWNV/1 -> Subsystem1/68(GW_StBttrySupplyVltMVBSWNV)
  GW_StBttrySupplyVltMVBSWErr/1 -> Subsystem1/67(GW_StBttrySupplyVltMVBSWErr)
  GW_BusTyp/1 -> Subsystem1/66(GW_BusTyp)
  GW_W_output/1 -> Subsystem1/65(GW_W_output)
  GW_StUvTopPrioErr/1 -> Subsystem1/64(GW_StUvTopPrioErr)
  Kitc_StKitcHostsSideSwtBotmNA/1 -> Subsystem1/63(Kitc_StKitcHostsSideSwtBotmNA)
  Kitc_StKitcHostsSideSwtBotmErr/1 -> Subsystem1/62(Kitc_StKitcHostsSideSwtBotmErr)
  Kitc_StKitcSwtBotmPartNA/1 -> Subsystem1/61(Kitc_StKitcSwtBotmPartNA)
  Kitc_StKitcSwtBotmPartErr/1 -> Subsystem1/60(Kitc_StKitcSwtBotmPartErr)
  Kitc_StKitcHostsSideSwtBotmPart/1 -> Subsystem1/59(Kitc_StKitcHostsSideSwtBotmPart)
  Kitc_StKitcHostsSideSwtUpprPart/1 -> Subsystem1/58(Kitc_StKitcHostsSideSwtUpprPart)
  Kitc_StKitcSwtUpprPart/1 -> Subsystem1/57(Kitc_StKitcSwtUpprPart)
  Kitc_TdOff/1 -> Subsystem1/56(Kitc_TdOff)
  Kitc_StDemoBd/1 -> Subsystem1/55(Kitc_StDemoBd)
  Toi_ToiInstlldInfo/1 -> Subsystem1/54(Toi_ToiInstlldInfo)
  GW_StClmpRdoOn/1 -> Subsystem1/53(GW_StClmpRdoOn)
  "GW_StEngAcvOn "/1 -> Subsystem1/52("GW_StEngAcvOn ")
  "Kitc_StTrfrSwt "/1 -> Subsystem1/51("Kitc_StTrfrSwt ")
  Kitc_StTrfrWoutNewStrt/1 -> Subsystem1/50(Kitc_StTrfrWoutNewStrt)
  Kitc_StTrfrBotmBtm/1 -> Subsystem1/49(Kitc_StTrfrBotmBtm)
  Kitc_StTrfrSwtTopBtn/1 -> Subsystem1/48(Kitc_StTrfrSwtTopBtn)
  Kitc_StTrfrSwtUpprPart/1 -> Subsystem1/47(Kitc_StTrfrSwtUpprPart)
  Kitc_TErrPuls/1 -> Subsystem1/46(Kitc_TErrPuls)
  Kitc_StsHostsCallAcvUpprDeck/1 -> Subsystem1/45(Kitc_StsHostsCallAcvUpprDeck)
  "GW_StClmp15On3SecOn "/1 -> Subsystem1/44("GW_StClmp15On3SecOn ")
  "GW_StrtLockOn "/1 -> Subsystem1/43("GW_StrtLockOn ")
  Kitc_StsWtrTankEmpty/1 -> Subsystem1/42(Kitc_StsWtrTankEmpty)
  Kitc_StHostsCallBlinkUpprDeck/1 -> Subsystem1/41(Kitc_StHostsCallBlinkUpprDeck)
  Kitc_StHostsCallBlink/1 -> Subsystem1/40(Kitc_StHostsCallBlink)
  "GW_StUvNormPrioOn "/1 -> Subsystem1/39("GW_StUvNormPrioOn ")
  Kitc_StsHostsCallAcv/1 -> Subsystem1/38(Kitc_StsHostsCallAcv)
  ABat_StAddlBatInstd/1 -> Subsystem1/37(ABat_StAddlBatInstd)
  GW_StEngRungOn/1 -> Subsystem1/36(GW_StEngRungOn)
  DBF_StsDoor1Open/1 -> Subsystem1/35(DBF_StsDoor1Open)
  GW_StClmp15On/1 -> Subsystem1/34(GW_StClmp15On)
  "GW_StStrtNewOn "/1 -> Subsystem1/33("GW_StStrtNewOn ")
  CLS_StDoorLockdOutd/1 -> Subsystem1/32(CLS_StDoorLockdOutd)
  Kitc_StKitcSwtUpprPartNA/1 -> Subsystem1/31(Kitc_StKitcSwtUpprPartNA)
  Kitc_StKitcSwtUpprPartErr/1 -> Subsystem1/30(Kitc_StKitcSwtUpprPartErr)
  Kitc_StKitcHostsSideSwtUpprNA/1 -> Subsystem1/29(Kitc_StKitcHostsSideSwtUpprNA)
  Kitc_StKitcHostsSideSwtUpprErr/1 -> Subsystem1/28(Kitc_StKitcHostsSideSwtUpprErr)
  Kitc_StTrfrSwtNA/1 -> Subsystem1/27(Kitc_StTrfrSwtNA)
  Kitc_StTrfrSwtErr/1 -> Subsystem1/26(Kitc_StTrfrSwtErr)
  Kitc_StTrfrBotmBtmNA/1 -> Subsystem1/25(Kitc_StTrfrBotmBtmNA)
  Kitc_StTrfrBotmBtmErr/1 -> Subsystem1/24(Kitc_StTrfrBotmBtmErr)
  Kitc_StTrfrSwtLowrPartNA/1 -> Subsystem1/23(Kitc_StTrfrSwtLowrPartNA)
  Kitc_StTrfrSwtLowrPartErr/1 -> Subsystem1/22(Kitc_StTrfrSwtLowrPartErr)
  Kitc_StTrfrSwtTopBtnNA/1 -> Subsystem1/21(Kitc_StTrfrSwtTopBtnNA)
  Kitc_StTrfrSwtTopBtnErr/1 -> Subsystem1/20(Kitc_StTrfrSwtTopBtnErr)
  Kitc_StTrfrSwtUpprPartNA/1 -> Subsystem1/19(Kitc_StTrfrSwtUpprPartNA)
  Kitc_StTrfrSwtUpprPartErr/1 -> Subsystem1/18(Kitc_StTrfrSwtUpprPartErr)
  GW_StEngAcvNV/1 -> Subsystem1/17(GW_StEngAcvNV)
  GW_StEngAcvErr/1 -> Subsystem1/16(GW_StEngAcvErr)
  GW_StClmpRdoNV/1 -> Subsystem1/15(GW_StClmpRdoNV)
  GW_StClmpRdoErr/1 -> Subsystem1/14(GW_StClmpRdoErr)
  GW_StClmp15On3SecErr/1 -> Subsystem1/13(GW_StClmp15On3SecErr)
  GW_StrtLockErr/1 -> Subsystem1/12(GW_StrtLockErr)
  GW_StUvNormPrioErr/1 -> Subsystem1/11(GW_StUvNormPrioErr)
  GW_StEngRungErr/1 -> Subsystem1/10(GW_StEngRungErr)
  GW_StClmp15Err/1 -> Subsystem1/9(GW_StClmp15Err)
  GW_StStrtNewErr/1 -> Subsystem1/8(GW_StStrtNewErr)
  GW_ModeExbnErr/1 -> Subsystem1/7(GW_ModeExbnErr)
  "GW_StBttrySupplyVltMVBSWOn "/1 -> Subsystem1/6("GW_StBttrySupplyVltMVBSWOn ")
  GW_SpdGrtr3/1 -> Subsystem1/5(GW_SpdGrtr3)
  "GW_ModeExbnOn "/1 -> Subsystem1/4("GW_ModeExbnOn ")
  "GW_StClmp50Off3Sec "/1 -> Subsystem1/3("GW_StClmp50Off3Sec ")
  GW_StUvLoPrio/1 -> Subsystem1/2(GW_StUvLoPrio)
  GW_StUvTopPrioOn/1 -> Subsystem1/1(GW_StUvTopPrioOn)
  Data Type Conversion/1 -> Switch/2
  Switch/1 -> Subsystem1/Enable
  Constant/1 -> Switch/3
  Data Store Read/1 -> Data Type Conversion/1, Switch/1

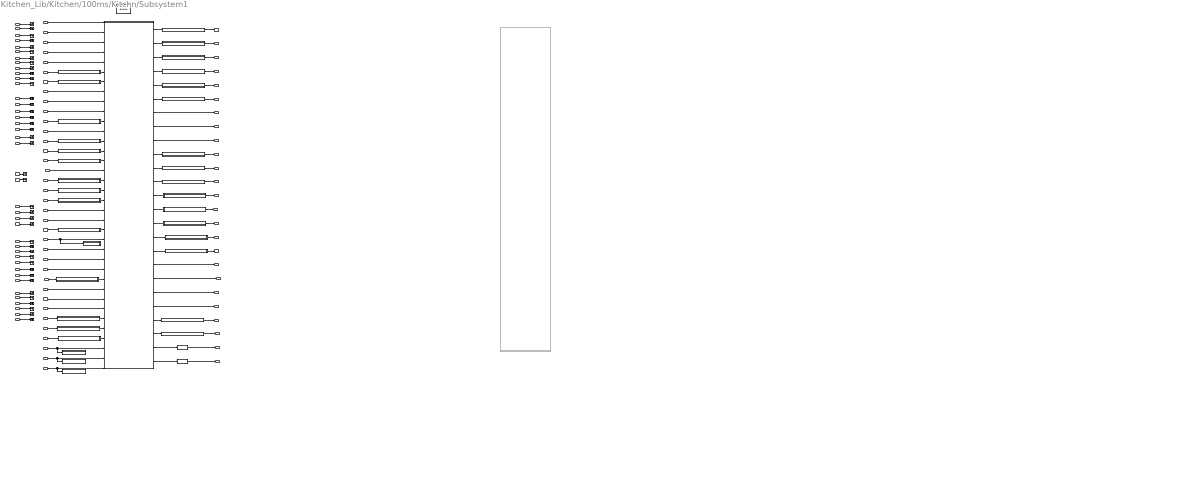
== system Kitchen_Lib/Kitchen/100ms/Kitchn/Subsystem1 ==
  note: Mustafa v1
  note: OLD MODEL
  GW_StUvTopPrioOn : Inport
  GW_StUvLoPrio : Inport  Port=2
  "GW_StClmp50Off3Sec " : Inport  Port=3
  "GW_ModeExbnOn " : Inport  Port=4
  GW_SpdGrtr3 : Inport  Port=5
  "GW_StBttrySupplyVltMVBSWOn " : Inport  Port=6
  GW_ModeExbnErr : Inport  Port=7
  GW_StStrtNewErr : Inport  Port=8
  GW_StClmp15Err : Inport  Port=9
  GW_StEngRungErr : Inport  Port=10
  GW_StUvNormPrioErr : Inport  Port=11
  GW_StrtLockErr : Inport  Port=12
  GW_StClmp15On3SecErr : Inport  Port=13
  GW_StClmpRdoErr : Inport  Port=14
  GW_StClmpRdoNV : Inport  Port=15
  GW_StEngAcvErr : Inport  Port=16
  GW_StEngAcvNV : Inport  Port=17
  Kitc_StTrfrSwtUpprPartErr : Inport  Port=18
  Kitc_StTrfrSwtUpprPartNA : Inport  Port=19
  Kitc_StTrfrSwtTopBtnErr : Inport  Port=20
  Kitc_StTrfrSwtTopBtnNA : Inport  Port=21
  Kitc_StTrfrSwtLowrPartErr : Inport  Port=22
  Kitc_StTrfrSwtLowrPartNA : Inport  Port=23
  Kitc_StTrfrBotmBtmErr : Inport  Port=24
  Kitc_StTrfrBotmBtmNA : Inport  Port=25
  Kitc_StTrfrSwtErr : Inport  Port=26
  Kitc_StTrfrSwtNA : Inport  Port=27
  Kitc_StKitcHostsSideSwtUpprErr : Inport  Port=28
  Kitc_StKitcHostsSideSwtUpprNA : Inport  Port=29
  Kitc_StKitcSwtUpprPartErr : Inport  Port=30
  Kitc_StKitcSwtUpprPartNA : Inport  Port=31
  CLS_StDoorLockdOutd : Inport  Port=32
  "GW_StStrtNewOn " : Inport  Port=33
  GW_StClmp15On : Inport  Port=34
  DBF_StsDoor1Open : Inport  Port=35
  GW_StEngRungOn : Inport  Port=36
  ABat_StAddlBatInstd : Inport  Port=37
  Kitc_StsHostsCallAcv : Inport  Port=38
  "GW_StUvNormPrioOn " : Inport  Port=39
  Kitc_StHostsCallBlink : Inport  Port=40
  Kitc_StHostsCallBlinkUpprDeck : Inport  Port=41
  Kitc_StsWtrTankEmpty : Inport  Port=42
  "GW_StrtLockOn " : Inport  Port=43
  "GW_StClmp15On3SecOn " : Inport  Port=44
  Kitc_StsHostsCallAcvUpprDeck : Inport  Port=45
  Kitc_TErrPuls : Inport  Port=46
  Kitc_StTrfrSwtUpprPart : Inport  Port=47
  Kitc_StTrfrSwtTopBtn : Inport  Port=48
  Kitc_StTrfrBotmBtm : Inport  Port=49
  Kitc_StTrfrWoutNewStrt : Inport  Port=50
  "Kitc_StTrfrSwt " : Inport  Port=51
  "GW_StEngAcvOn " : Inport  Port=52
  GW_StClmpRdoOn : Inport  Port=53
  Toi_ToiInstlldInfo : Inport  Port=54
  Kitc_StDemoBd : Inport  Port=55
  Kitc_TdOff : Inport  Port=56
  Kitc_StKitcSwtUpprPart : Inport  Port=57
  Kitc_StKitcHostsSideSwtUpprPart : Inport  Port=58
  Kitc_StKitcHostsSideSwtBotmPart : Inport  Port=59
  Kitc_StKitcSwtBotmPartErr : Inport  Port=60
  Kitc_StKitcSwtBotmPartNA : Inport  Port=61
  Kitc_StKitcHostsSideSwtBotmErr : Inport  Port=62
  Kitc_StKitcHostsSideSwtBotmNA : Inport  Port=63
  GW_StUvTopPrioErr : Inport  Port=64
  GW_W_output : Inport  Port=65
  GW_BusTyp : Inport  Port=66
  GW_StBttrySupplyVltMVBSWErr : Inport  Port=67
  GW_StBttrySupplyVltMVBSWNV : Inport  Port=68
  Enable : EnablePort
  Data Type Conversion : DataTypeConversion  OutDataTypeStr=uint8  SaturateOnIntegerOverflow=off  RndMeth=Floor
  Data Type Conversion1 : DataTypeConversion  OutDataTypeStr=uint8  SaturateOnIntegerOverflow=off  RndMeth=Floor
  GW_ModeExbnNV : InportShadow  Port=7
  GW_StClmp15NV : InportShadow  Port=9
  GW_StClmp15On3SecNV : InportShadow  Port=13
  GW_StEngRungNV : InportShadow  Port=10
  GW_StStrtNewNV : InportShadow  Port=8
  GW_StUvNormPrioNV : InportShadow  Port=11
  GW_StUvTopPrioNV : InportShadow  Port=64
  GW_StrtLockNV : InportShadow  Port=12
  Subsystem1 : Subsystem
  Subsystem10 : Subsystem
  Subsystem11 : Subsystem
  Subsystem12 : Subsystem
  Subsystem13 : Subsystem
  Subsystem14 : Subsystem
  Subsystem15 : Subsystem
  Subsystem16 : Subsystem  Commented=on
  Subsystem17 : Subsystem
  Subsystem19 : Subsystem
  Subsystem2 : Subsystem
  Subsystem20 : Subsystem
  Subsystem21 : Subsystem
  Subsystem22 : Subsystem
  Subsystem23 : Subsystem
  Subsystem24 : Subsystem
  Subsystem25 : Subsystem
  Subsystem26 : Subsystem
  Subsystem27 : Subsystem
  Subsystem28 : Subsystem
  Subsystem29 : Subsystem
  Subsystem3 : Subsystem
  Subsystem30 : Subsystem
  Subsystem31 : Subsystem
  Subsystem32 : Subsystem
  Subsystem33 : Subsystem
  Subsystem34 : Subsystem
  Subsystem35 : Subsystem
  Subsystem36 : Subsystem
  Subsystem4 : Subsystem
  Subsystem41 : Subsystem
  Subsystem5 : Subsystem
  Subsystem6 : Subsystem
  Subsystem7 : Subsystem
  Subsystem8 : Subsystem
  Subsystem9 : Subsystem
  Terminator{,1..39} (40 alike) : Terminator
  Kitc_StsKitcAcv : Outport
  Kitc_StBuzRe : Outport  Port=2
  Kitc_StLrgCns : Outport  Port=3
  Kitc_StSmlCns : Outport  Port=4
  Kitc_StsPwmFreq : Outport  Port=5
  Kitc_StTrfr : Outport  Port=6
  Kitc_TrfrSwtLed : Outport  Port=7
  Kitc_KitcHostsSideSwtLed : Outport  Port=8
  Kitc_KitcSwtLed : Outport  Port=9
  Kitc_EidWtrTankEmpty : Outport  Port=10
  Kitc_StRefgtr : Outport  Port=11
  Kitc_StHostsCall : Outport  Port=12
  Kitchn_StAcvCode : Outport  Port=13
  Kitc_StTrfrInstd : Outport  Port=14
  "Kitc_StFrntRefgtr " : Outport  Port=15
  Kitc_PwmHostsCall : Outport  Port=16
  Kitc_KtchnLowBttryNotRlsd : Outport  Port=17
  Kitc_KitchenReleased : Outport  Port=18
  Kitc_KitchenNotReleased : Outport  Port=19
  Kitc_StsPwmFreq2 : Outport  Port=20
  Kitc_AcvSkyliner : Outport  Port=21
  Kitc_ShtdwnReqPermsn : Outport  Port=22
  Kitc_ShtdwnReqBlck : Outport  Port=23
  Kitch_dispWtrTnkLvlWrng : Outport  Port=24
  Kitch_dispKitchenPssngrReqAcv : Outport  Port=25
  wires:
  Data Type Conversion1/1 -> Kitch_dispKitchenPssngrReqAcv/1
  Data Type Conversion/1 -> Kitch_dispWtrTnkLvlWrng/1
  Subsystem19/25(Kitch_dispKitchenPssngrReqAcv) -> Data Type Conversion1/1
  Subsystem19/24(Kitch_dispWtrTnkLvlWrng) -> Data Type Conversion/1
  Subsystem19/21(Kitc_ShtdwnReqBlck) -> Kitc_ShtdwnReqBlck/1
  Subsystem19/20(Kitc_ShtdwnReqPermsn) -> Kitc_ShtdwnReqPermsn/1
  Subsystem19/19(Kitc_AcvSkyliner) -> Kitc_AcvSkyliner/1
  Subsystem19/18(Kitc_StsPwmFreq2) -> Kitc_StsPwmFreq2/1
  GW_StrtLockErr/1 -> Terminator10/1
  GW_StUvNormPrioNV/1 -> Terminator9/1
  GW_StUvNormPrioErr/1 -> Terminator8/1
  GW_StEngRungNV/1 -> Terminator7/1
  GW_StEngRungErr/1 -> Terminator6/1
  Subsystem13/1(DBF_StsDoor1Open_E2E) -> Subsystem19/11(DBF_StsDoor1Open)
  Subsystem9/1(Kitc_StTrfrWoutNewStrt_E2E) -> Subsystem19/27(Kitc_StTrfrWoutNewStrt)
  Kitc_StKitcSwtUpprPart/1 -> Subsystem19/1(Kitc_StKitcSwtUpprPart)
  Kitc_StKitcHostsSideSwtUpprPart/1 -> Subsystem19/2(Kitc_StKitcHostsSideSwtUpprPart)
  Kitc_StKitcHostsSideSwtBotmPart/1 -> Subsystem19/3(Kitc_StKitcHostsSideSwtBotmPart)
  Subsystem36/1(CLS_StDoorLockdOutd_E2E) -> Subsystem19/7(CLS_StDoorLockdOutd)
  Subsystem35/1(LRL_StLggRoomRiLi_Frq_E2E) -> Kitc_PwmHostsCall/1
  Subsystem34/1(Kitchn_StAcvCode_E2E) -> Kitchn_StAcvCode/1
  Subsystem33/1(Kitc_StHostsCall_E2E) -> Kitc_StHostsCall/1
  Subsystem32/1(LRL_StOverHdLggRiLi_E2E) -> Kitc_KitchenNotReleased/1
  Subsystem31/1(LRL_StOverHdLggRiLi_E2E) -> Kitc_KitchenReleased/1
  Subsystem30/1(LRL_StOverHdLggRiLi_E2E) -> Kitc_KtchnLowBttryNotRlsd/1
  Subsystem29/1(LRL_StOverHdLggRiLi_E2E) -> "Kitc_StFrntRefgtr "/1
  Subsystem28/1(Kitc_StTrfrInstd_E2E) -> Kitc_StTrfrInstd/1
  Subsystem27/1(Kitc_StRefgtr_E2E) -> Kitc_StRefgtr/1
  Subsystem26/1(Kitc_EidWtrTankEmpty_E2E) -> Kitc_EidWtrTankEmpty/1
  Subsystem24/1(Kitc_StTrfr_E2E) -> Kitc_StTrfr/1
  Subsystem23/1(Kitc_StsPwmFreq_E2E) -> Kitc_StsPwmFreq/1
  Subsystem22/1(Kitc_StSmlCns_E2E) -> Kitc_StSmlCns/1
  Subsystem41/1(Kitc_StLrgCns_E2E) -> Kitc_StLrgCns/1
  Subsystem21/1(Kitc_StBuzRe_E2E) -> Kitc_StBuzRe/1
  Subsystem25/1(Kitc_StsKitcAcv_E2E) -> Kitc_StsKitcAcv/1
  Subsystem15/1(Kitc_StDemoBd_E2E) -> Subsystem19/33(Kitc_StDemoBd)
  Subsystem14/1(Toi_ToiInstlldInfo_E2E) -> Subsystem19/32(Toi_ToiInstlldInfo)
  "Kitc_StTrfrSwt "/1 -> Subsystem19/28("Kitc_StTrfrSwt ")
  Kitc_StTrfrWoutNewStrt/1 -> Subsystem9/1(Kitc_StTrfrWoutNewStrt)
  Kitc_StTrfrBotmBtm/1 -> Subsystem19/26(Kitc_StTrfrBotmBtm)
  Kitc_StTrfrSwtUpprPart/1 -> Subsystem19/24(Kitc_StTrfrSwtUpprPart)
  Subsystem8/1(Kitc_StsHostsCallAcvUpprDeck_E2E) -> Subsystem19/22(Kitc_StsHostsCallAcvUpprDeck)
  Subsystem6/1(Kitc_StsWtrTankEmpty_E2E) -> Subsystem19/19(Kitc_StsWtrTankEmpty)
  Subsystem4/1(Kitc_StHostsCallBlinkUpprDeck_E2E) -> Subsystem19/18(Kitc_StHostsCallBlinkUpprDeck)
  Subsystem3/1(Kitc_StHostsCallBlink_E2E) -> Subsystem19/17(Kitc_StHostsCallBlink)
  Subsystem2/1(ABat_StAddlBatInstd_E2E) -> Subsystem19/13(ABat_StAddlBatInstd)
  Subsystem1/1(Kitc_StsHostsCallAcv_E2E) -> Subsystem19/14(Kitc_StsHostsCallAcv)
  GW_StBttrySupplyVltMVBSWNV/1 -> Terminator39/1
  GW_StBttrySupplyVltMVBSWErr/1 -> Terminator38/1
  GW_BusTyp/1 -> Subsystem11/1(GW_BusTyp), Subsystem19/36(GW_BusTyp)
  Subsystem19/23(Kitc_KitchenNotReleased) -> Subsystem32/1(LRL_StOverHdLggRiLi)
  Subsystem19/22(Kitc_KitchenReleased) -> Subsystem31/1(LRL_StOverHdLggRiLi)
  Subsystem19/17(Kitc_KtchnLowBttryNotRlsd) -> Subsystem30/1(LRL_StOverHdLggRiLi)
  Subsystem19/16(Kitc_PwmHostsCall) -> Subsystem35/1(LRL_StLggRoomRiLi_Frq)
  Subsystem19/15("Kitc_StFrntRefgtr ") -> Subsystem29/1(LRL_StOverHdLggRiLi)
  Subsystem19/14(Kitc_StTrfrInstd) -> Subsystem28/1(Kitc_StTrfrInstd)
  Subsystem19/13(Kitchn_StAcvCode) -> Subsystem34/1(Kitchn_StAcvCode)
  Subsystem19/12(Kitc_StHostsCall) -> Subsystem33/1(Kitc_StHostsCall)
  Subsystem19/11(Kitc_StRefgtr) -> Subsystem27/1(Kitc_StRefgtr)
  Subsystem19/10(Kitc_EidWtrTankEmpty) -> Subsystem26/1(Kitc_EidWtrTankEmpty)
  Subsystem19/9(Kitc_KitcSwtLed) -> Kitc_KitcSwtLed/1
  Subsystem19/8(Kitc_KitcHostsSideSwtLed) -> Kitc_KitcHostsSideSwtLed/1
  Subsystem19/7(Kitc_TrfrSwtLed) -> Kitc_TrfrSwtLed/1
  Subsystem19/6(Kitc_StTrfr) -> Subsystem24/1(Kitc_StTrfr)
  Subsystem19/5(Kitc_StsPwmFreq) -> Subsystem23/1(Kitc_StsPwmFreq)
  Subsystem19/4(Kitc_StSmlCns) -> Subsystem22/1(Kitc_StSmlCns)
  Subsystem19/3(Kitc_StLrgCns) -> Subsystem41/1(Kitc_StLrgCns)
  Subsystem19/2(Kitc_StBuzRe) -> Subsystem21/1(Kitc_StBuzRe)
  Subsystem19/1(Kitc_StsKitcAcv) -> Subsystem25/1(Kitc_StsKitcAcv)
  GW_W_output/1 -> Subsystem19/35(GW_W_output), Subsystem10/1(GW_W_output)
  GW_StUvTopPrioNV/1 -> Terminator37/1
  GW_StUvTopPrioErr/1 -> Terminator36/1
  Kitc_StKitcHostsSideSwtBotmNA/1 -> Terminator35/1
  Kitc_StKitcHostsSideSwtBotmErr/1 -> Terminator34/1
  Kitc_StKitcSwtBotmPartNA/1 -> Terminator33/1
  Kitc_StKitcSwtBotmPartErr/1 -> Terminator32/1
  Kitc_TdOff/1 -> Subsystem19/34(Kitc_TdOff), Subsystem17/1(Kitc_TdOff_E2E)
  Kitc_StDemoBd/1 -> Subsystem15/1(Kitc_StDemoBd)
  Toi_ToiInstlldInfo/1 -> Subsystem14/1(Toi_ToiInstlldInfo)
  GW_StClmpRdoOn/1 -> Subsystem19/30(GW_StClmpRdo)
  "GW_StEngAcvOn "/1 -> Subsystem19/29("GW_StEngAcv ")
  Kitc_StTrfrSwtTopBtn/1 -> Subsystem19/25(Kitc_StTrfrSwtTopBtn)
  Kitc_TErrPuls/1 -> Subsystem19/23(Kitc_TErrPuls), Subsystem20/1(Kitc_TErrPuls_E2E)
  Kitc_StsHostsCallAcvUpprDeck/1 -> Subsystem8/1(Kitc_StsHostsCallAcvUpprDeck)
  "GW_StClmp15On3SecOn "/1 -> Subsystem19/21("GW_StClmp15On3Sec ")
  "GW_StrtLockOn "/1 -> Subsystem19/20("GW_StrtLock ")
  Kitc_StsWtrTankEmpty/1 -> Subsystem6/1(Kitc_StsWtrTankEmpty)
  Kitc_StHostsCallBlinkUpprDeck/1 -> Subsystem4/1(Kitc_StHostsCallBlinkUpprDeck)
  Kitc_StHostsCallBlink/1 -> Subsystem3/1(Kitc_StHostsCallBlink)
  "GW_StUvNormPrioOn "/1 -> Subsystem19/16("GW_StUvNormPrio ")
  Kitc_StsHostsCallAcv/1 -> Subsystem1/1(Kitc_StsHostsCallAcv)
  ABat_StAddlBatInstd/1 -> Subsystem2/1(ABat_StAddlBatInstd)
  GW_StEngRungOn/1 -> Subsystem19/12(GW_StEngRung)
  DBF_StsDoor1Open/1 -> Subsystem13/1(DBF_StsDoor1Open)
  GW_StClmp15On/1 -> Subsystem19/10(GW_StClmp15)
  "GW_StStrtNewOn "/1 -> Subsystem19/8("GW_StStrtNew ")
  CLS_StDoorLockdOutd/1 -> Subsystem36/1(CLS_StDoorLockdOutd)
  Subsystem5/1(GW_StUvLoPrio_E2E) -> Subsystem19/31("GW_StUvLoPrio ")
  Subsystem7/1(GW_StClmp50Off3Sec_E2E) -> Subsystem19/15("GW_StClmp50Off3Sec ")
  Subsystem12/1(GW_SpdGrtr3_E2E) -> Subsystem19/6(GW_SpdGrtr3)
  "GW_ModeExbnOn "/1 -> Subsystem19/5("GW_ModeExbn ")
  Kitc_StKitcSwtUpprPartNA/1 -> Terminator21/1
  Kitc_StKitcSwtUpprPartErr/1 -> Terminator20/1
  Kitc_StKitcHostsSideSwtUpprNA/1 -> Terminator23/1
  Kitc_StKitcHostsSideSwtUpprErr/1 -> Terminator22/1
  Kitc_StTrfrSwtNA/1 -> Terminator31/1
  Kitc_StTrfrSwtErr/1 -> Terminator30/1
  Kitc_StTrfrBotmBtmNA/1 -> Terminator29/1
  Kitc_StTrfrBotmBtmErr/1 -> Terminator28/1
  Kitc_StTrfrSwtLowrPartNA/1 -> Terminator27/1
  Kitc_StTrfrSwtLowrPartErr/1 -> Terminator26/1
  Kitc_StTrfrSwtTopBtnNA/1 -> Terminator25/1
  Kitc_StTrfrSwtTopBtnErr/1 -> Terminator24/1
  Kitc_StTrfrSwtUpprPartNA/1 -> Terminator19/1
  Kitc_StTrfrSwtUpprPartErr/1 -> Terminator18/1
  GW_StEngAcvNV/1 -> Terminator17/1
  GW_StEngAcvErr/1 -> Terminator16/1
  GW_StClmpRdoNV/1 -> Terminator15/1
  GW_StClmpRdoErr/1 -> Terminator14/1
  GW_StClmp15On3SecNV/1 -> Terminator13/1
  GW_StClmp15On3SecErr/1 -> Terminator12/1
  GW_StrtLockNV/1 -> Terminator11/1
  GW_StClmp15NV/1 -> Terminator5/1
  GW_StClmp15Err/1 -> Terminator4/1
  GW_StStrtNewNV/1 -> Terminator3/1
  GW_StStrtNewErr/1 -> Terminator2/1
  GW_ModeExbnNV/1 -> Terminator1/1
  GW_ModeExbnErr/1 -> Terminator/1
  GW_StUvTopPrioOn/1 -> Subsystem19/9(GW_StUvTopPrio)
  "GW_StBttrySupplyVltMVBSWOn "/1 -> Subsystem19/4(GW_StBttrySupplyVltMVBSWOn)
  GW_SpdGrtr3/1 -> Subsystem12/1(GW_SpdGrtr3)
  "GW_StClmp50Off3Sec "/1 -> Subsystem7/1(GW_StClmp50Off3Sec)
  GW_StUvLoPrio/1 -> Subsystem5/1(GW_StUvLoPrio)
